simulink model "mrefrobotarm_previous_y_previous_u_previous_ref_cex_3b"  (R2018b)
settings: Solver=FixedStepAuto  StartTime=0.0  StopTime=20  RelTol=1e-3  AbsTol=1e-6
undefined symbols (not defined in the file or in its folder): cc, options
libraries: neural x462, simulink x2
(part 16 of 18)

== system mrefrobotarm_previous_y_previous_u_previous_ref_cex_3b/no_cex/Layer 3/Delays 1 ==
  "p{3}" : Inport  PortDimensions=30
      mask Display: e = 0.06;c1 = [120 230 180]/255;c2 = ([120 230 180]+0)/(256+128);c3 = ([120 230 180]+128)/(256+128);patch([0 1 1 0],[0 0 1 1],c1);patch([0 1 1 1-e 1-e 0+e],[0 0 1 1-e 0+e 0+e],c2);patch([0 0 1 1-e 0+e 0+e],[0 1 1 1-e 1-e 0+e],c3);plot([0 1 1 0 0],[0 0 1 1 0]);
  mux : Mux  Inputs=1
      mask Display: e = 0.06;c1 = [120 150 230]/255;c2 = ([120 150 230]+0)/383;c3 = ([120 150 230]+128)/383;patch([0 1 1 0],[0 0 1 1],c1);patch([0 1 1 1-e 1-e 0+e],[0 0 1 1-e 0+e 0+e],c2);patch([0 0 1 1-e 0+e 0+e],[0 1 1 1-e 1-e 0+e],c3);plot([0 1 1 0 0],[0 0 1 1 0]);disp('Mux')
  "pd{3,2}" : Outport
      mask Display: e = 0.06;c1 = [120 230 180]/255;c2 = ([120 230 180]+0)/(256+128);c3 = ([120 230 180]+128)/(256+128);patch([0 1 1 0],[0 0 1 1],c1);patch([0 1 1 1-e 1-e 0+e],[0 0 1 1-e 0+e 0+e],c2);patch([0 0 1 1-e 0+e 0+e],[0 1 1 1-e 1-e 0+e],c3);plot([0 1 1 0 0],[0 0 1 1 0]);
  wires:
  "p{3}"/1 -> mux/1
  mux/1 -> "pd{3,2}"/1

== system mrefrobotarm_previous_y_previous_u_previous_ref_cex_3b/no_cex/Layer 3/LW{3,2} ==
  "ad{3,2}" : Inport  PortDimensions=30
      mask Display: e = 0.06;c1 = [120 230 180]/255;c2 = ([120 230 180]+0)/(256+128);c3 = ([120 230 180]+128)/(256+128);patch([0 1 1 0],[0 0 1 1],c1);patch([0 1 1 1-e 1-e 0+e],[0 0 1 1-e 0+e 0+e],c2);patch([0 0 1 1-e 0+e 0+e],[0 1 1 1-e 1-e 0+e],c3);plot([0 1 1 0 0],[0 0 1 1 0]);
  "IW{3,2}(1,:)'" : Constant  Value=[-0.055044119527404726521790934157252195291221141815185546875;-0.328920591070812451395255493480362929403781890869140625;0.415372619414880739352469163350178860127925872802734375;-0.228280394241074768846289089196943677961826324462890625;0.16685877262507620155673748740809969604015350341796875;-0.28767716315785907266189269648748449981212615966796875;-0.32128097238228281451455359274405054748058319091796875;0.1207208021741804360171812504631816409528255462646484375;-0.01460580260399220453582103118606028147041797637939453125;0.50165908559916350117902084093657322227954864501953125;0.35772322215377549969872461588238365948200225830078125;-0.00629781978787156970778227105256519280374050140380859375;-0.045079348120089589302406096749109565280377864837646484375;0.00997084703321709196754962789555065683089196681976318359375;0.28527054426915376961204628969426266849040985107421875;0.249132491312471116007287719185114838182926177978515625;-0.1838303477417790876558001400553621351718902587890625;0.4598700488107703154838645787094719707965850830078125;0.0369702760794284046586000158640672452747821807861328125;0.038819346858363877605935243764179176650941371917724609375;0.3202062144887756200972717124386690557003021240234375;-0.022206955571550758554710824910216615535318851470947265625;0.1764209554328330098460497765699983574450016021728515625;-0.369049855517247060721075513356481678783893585205078125;-0.0296667490766724904760476277942871092818677425384521484375;-0.0365536479267042080376626245197257958352565765380859375;0.278066415559107327215571103806723840534687042236328125;0.55989740946528510079360785312019288539886474609375;-0.217843605833106190861059303642832674086093902587890625;0.4063996140330810025176333510898984968662261962890625]
      mask Display: e = 0.06;c1 = [120 150 230]/255;c2 = ([120 150 230]+0)/383;c3 = ([120 150 230]+128)/383;patch([0 1 1 0],[0 0 1 1],c1);patch([0 1 1 1-e 1-e 0+e],[0 0 1 1-e 0+e 0+e],c2);patch([0 0 1 1-e 0+e 0+e],[0 1 1 1-e 1-e 0+e],c3);plot([0 1 1 0 0],[0 0 1 1 0]);disp('weights');
  Mux : Mux  Inputs=1
      mask Display: e = 0.06;c1 = [120 150 230]/255;c2 = ([120 150 230]+0)/383;c3 = ([120 150 230]+128)/383;patch([0 1 1 0],[0 0 1 1],c1);patch([0 1 1 1-e 1-e 0+e],[0 0 1 1-e 0+e 0+e],c2);patch([0 0 1 1-e 0+e 0+e],[0 1 1 1-e 1-e 0+e],c3);plot([0 1 1 0 0],[0 0 1 1 0]);disp('Mux');
  dotprod1 : neural/Weight Functions/dotprod
  "lz{3,2}" : Outport
      mask Display: e = 0.06;c1 = [120 230 180]/255;c2 = ([120 230 180]+0)/(256+128);c3 = ([120 230 180]+128)/(256+128);patch([0 1 1 0],[0 0 1 1],c1);patch([0 1 1 1-e 1-e 0+e],[0 0 1 1-e 0+e 0+e],c2);patch([0 0 1 1-e 0+e 0+e],[0 1 1 1-e 1-e 0+e],c3);plot([0 1 1 0 0],[0 0 1 1 0]);
  wires:
  "IW{3,2}(1,:)'"/1 -> dotprod1/1
  "ad{3,2}"/1 -> dotprod1/2
  dotprod1/1 -> Mux/1
  Mux/1 -> "lz{3,2}"/1

== system mrefrobotarm_previous_y_previous_u_previous_ref_cex_3b/no_cex_15000/Layer 1/Delays 1 ==
  "p{1}" : Inport  PortDimensions=10
      mask Display: e = 0.06;c1 = [120 230 180]/255;c2 = ([120 230 180]+0)/(256+128);c3 = ([120 230 180]+128)/(256+128);patch([0 1 1 0],[0 0 1 1],c1);patch([0 1 1 1-e 1-e 0+e],[0 0 1 1-e 0+e 0+e],c2);patch([0 0 1 1-e 0+e 0+e],[0 1 1 1-e 1-e 0+e],c3);plot([0 1 1 0 0],[0 0 1 1 0]);
  mux : Mux  Inputs=1
      mask Display: e = 0.06;c1 = [120 150 230]/255;c2 = ([120 150 230]+0)/383;c3 = ([120 150 230]+128)/383;patch([0 1 1 0],[0 0 1 1],c1);patch([0 1 1 1-e 1-e 0+e],[0 0 1 1-e 0+e 0+e],c2);patch([0 0 1 1-e 0+e 0+e],[0 1 1 1-e 1-e 0+e],c3);plot([0 1 1 0 0],[0 0 1 1 0]);disp('Mux')
  "pd{1,1}" : Outport
      mask Display: e = 0.06;c1 = [120 230 180]/255;c2 = ([120 230 180]+0)/(256+128);c3 = ([120 230 180]+128)/(256+128);patch([0 1 1 0],[0 0 1 1],c1);patch([0 1 1 1-e 1-e 0+e],[0 0 1 1-e 0+e 0+e],c2);patch([0 0 1 1-e 0+e 0+e],[0 1 1 1-e 1-e 0+e],c3);plot([0 1 1 0 0],[0 0 1 1 0]);
  wires:
  "p{1}"/1 -> mux/1
  mux/1 -> "pd{1,1}"/1

== system mrefrobotarm_previous_y_previous_u_previous_ref_cex_3b/no_cex_15000/Layer 1/IW{1,1} ==
  "pd{1,1}" : Inport  PortDimensions=10
      mask Display: e = 0.06;c1 = [120 230 180]/255;c2 = ([120 230 180]+0)/(256+128);c3 = ([120 230 180]+128)/(256+128);patch([0 1 1 0],[0 0 1 1],c1);patch([0 1 1 1-e 1-e 0+e],[0 0 1 1-e 0+e 0+e],c2);patch([0 0 1 1-e 0+e 0+e],[0 1 1 1-e 1-e 0+e],c3);plot([0 1 1 0 0],[0 0 1 1 0]);
  "IW{1,1}(1,:)'" : Constant  Value=[1.3188511834995317872909481593524105846881866455078125;0.1689480064871527187353450472073745913803577423095703125;0.62298389676086063371229784024762921035289764404296875;-0.39415218427752141128195262353983707726001739501953125;-1.5063673389761664811459240809199400246143341064453125;0.50937741333875352633953070835559628903865814208984375;0.32241543481989853869862372448551468551158905029296875;-0.335387271762626670845719445424037985503673553466796875;-0.58355235109725145381531774546601809561252593994140625;-0.7762464783952396363275738622178323566913604736328125]
      mask Display: e = 0.06;c1 = [120 150 230]/255;c2 = ([120 150 230]+0)/383;c3 = ([120 150 230]+128)/383;patch([0 1 1 0],[0 0 1 1],c1);patch([0 1 1 1-e 1-e 0+e],[0 0 1 1-e 0+e 0+e],c2);patch([0 0 1 1-e 0+e 0+e],[0 1 1 1-e 1-e 0+e],c3);plot([0 1 1 0 0],[0 0 1 1 0]);disp('Weights');
  "IW{1,1}(10,:)'" : Constant  Value=[0.7258859937732449196801098878495395183563232421875;0.2198238550287085202317172161201597191393375396728515625;-0.8129477677772023458402372853015549480915069580078125;0.33409670991292717001641676688450388610363006591796875;0.0762009301501332669825927723650238476693630218505859375;-0.82337222475456883774569405431975610554218292236328125;-0.2019297950314020706485962364240549504756927490234375;-0.88894889200459825673306113458238542079925537109375;2.436157192480757682773173655732534825801849365234375;1.0058276487454878012073322679498232901096343994140625]
      mask Display: e = 0.06;c1 = [120 150 230]/255;c2 = ([120 150 230]+0)/383;c3 = ([120 150 230]+128)/383;patch([0 1 1 0],[0 0 1 1],c1);patch([0 1 1 1-e 1-e 0+e],[0 0 1 1-e 0+e 0+e],c2);patch([0 0 1 1-e 0+e 0+e],[0 1 1 1-e 1-e 0+e],c3);plot([0 1 1 0 0],[0 0 1 1 0]);disp('Weights');
  "IW{1,1}(11,:)'" : Constant  Value=[-0.329810980731012393096790447089006192982196807861328125;0.4709000776860030601511653003399260342121124267578125;-0.98003410643667676627188711790950037539005279541015625;-0.87082647230757237455378572121844626963138580322265625;0.277016665627538072325108942095539532601833343505859375;-0.62337730541465308231607878042268566787242889404296875;0.7378401075831104716229447149089537560939788818359375;-0.436280563315827374371025371146970428526401519775390625;-0.6186629749781584752810204008710570633411407470703125;-0.7776858363996261847006508105550892651081085205078125]
      mask Display: e = 0.06;c1 = [120 150 230]/255;c2 = ([120 150 230]+0)/383;c3 = ([120 150 230]+128)/383;patch([0 1 1 0],[0 0 1 1],c1);patch([0 1 1 1-e 1-e 0+e],[0 0 1 1-e 0+e 0+e],c2);patch([0 0 1 1-e 0+e 0+e],[0 1 1 1-e 1-e 0+e],c3);plot([0 1 1 0 0],[0 0 1 1 0]);disp('Weights');
  "IW{1,1}(12,:)'" : Constant  Value=[0.53957951436292883595768898885580711066722869873046875;-0.55367319387039370948144778594723902642726898193359375;-1.067806415094755490002853548503480851650238037109375;-0.314790535031305107604993054337683133780956268310546875;-0.0301903113325120535381795860985221224837005138397216796875;-0.79597972460447252718296340390224941074848175048828125;0.9233408613690290422937323455698788166046142578125;0.28002836652928431160347599870874546468257904052734375;-0.612473068190372060826121014542877674102783203125;0.15412925045282188651896149167441762983798980712890625]
      mask Display: e = 0.06;c1 = [120 150 230]/255;c2 = ([120 150 230]+0)/383;c3 = ([120 150 230]+128)/383;patch([0 1 1 0],[0 0 1 1],c1);patch([0 1 1 1-e 1-e 0+e],[0 0 1 1-e 0+e 0+e],c2);patch([0 0 1 1-e 0+e 0+e],[0 1 1 1-e 1-e 0+e],c3);plot([0 1 1 0 0],[0 0 1 1 0]);disp('Weights');
  "IW{1,1}(13,:)'" : Constant  Value=[-0.007549105306197079374996850020806959946639835834503173828125;0.59264210166261055423575498934951610863208770751953125;-1.1503522427627166369035194293246604502201080322265625;0.462568606233602130917148542721406556665897369384765625;-0.17257805815617188738286813531885854899883270263671875;0.64446689676790158696206844979315064847469329833984375;-0.1690380289985726758317241547047160565853118896484375;-0.55825379012550324642205623604240827262401580810546875;-1.313955467045924141444857013993896543979644775390625;-0.76754440805176094020367827397421933710575103759765625]
      mask Display: e = 0.06;c1 = [120 150 230]/255;c2 = ([120 150 230]+0)/383;c3 = ([120 150 230]+128)/383;patch([0 1 1 0],[0 0 1 1],c1);patch([0 1 1 1-e 1-e 0+e],[0 0 1 1-e 0+e 0+e],c2);patch([0 0 1 1-e 0+e 0+e],[0 1 1 1-e 1-e 0+e],c3);plot([0 1 1 0 0],[0 0 1 1 0]);disp('Weights');
  "IW{1,1}(14,:)'" : Constant  Value=[0.28879437950909914167851866295677609741687774658203125;0.309031337007359019342089823112473823130130767822265625;0.35490953690414117627227597040473483502864837646484375;0.44617557915201933038673587361699901521205902099609375;-0.817158931264831966956307951477356255054473876953125;-0.631792498376267275261852773837745189666748046875;-0.78411392315008521247676753773703239858150482177734375;0.57409330632700716900984616586356423795223236083984375;0.78284637315219562925250329499249346554279327392578125;-1.07999096319560639045675998204387724399566650390625]
      mask Display: e = 0.06;c1 = [120 150 230]/255;c2 = ([120 150 230]+0)/383;c3 = ([120 150 230]+128)/383;patch([0 1 1 0],[0 0 1 1],c1);patch([0 1 1 1-e 1-e 0+e],[0 0 1 1-e 0+e 0+e],c2);patch([0 0 1 1-e 0+e 0+e],[0 1 1 1-e 1-e 0+e],c3);plot([0 1 1 0 0],[0 0 1 1 0]);disp('Weights');
  "IW{1,1}(15,:)'" : Constant  Value=[-0.2265915888454878845958972988228197209537029266357421875;0.52512734507735758793245395281701348721981048583984375;-0.237067451495421244178629649468348361551761627197265625;-0.50711573329694614731266710805357433855533599853515625;0.53852671039054500479181797345518134534358978271484375;-0.58079797081326611785101476925774477422237396240234375;0.995671396692161092545347855775617063045501708984375;-0.93945924504259947784845508067519403994083404541015625;-1.025726388686293066854204880655743181705474853515625;-0.38905464320706872882738025509752333164215087890625]
      mask Display: e = 0.06;c1 = [120 150 230]/255;c2 = ([120 150 230]+0)/383;c3 = ([120 150 230]+128)/383;patch([0 1 1 0],[0 0 1 1],c1);patch([0 1 1 1-e 1-e 0+e],[0 0 1 1-e 0+e 0+e],c2);patch([0 0 1 1-e 0+e 0+e],[0 1 1 1-e 1-e 0+e],c3);plot([0 1 1 0 0],[0 0 1 1 0]);disp('Weights');
  "IW{1,1}(16,:)'" : Constant  Value=[-0.0999221466547733638829953406457207165658473968505859375;0.58666448347591571010894995197304524481296539306640625;0.38727263657233290672365910722874104976654052734375;-1.063470901218607878035982139408588409423828125;-0.51664598743441902950479516221093945205211639404296875;0.2823348550820128366467542946338653564453125;1.1755784087792588987753106266609393060207366943359375;-0.3872581958704384152980537692201323807239532470703125;-1.157082121110430517063605293515138328075408935546875;-0.139943189411582846748416386617464013397693634033203125]
      mask Display: e = 0.06;c1 = [120 150 230]/255;c2 = ([120 150 230]+0)/383;c3 = ([120 150 230]+128)/383;patch([0 1 1 0],[0 0 1 1],c1);patch([0 1 1 1-e 1-e 0+e],[0 0 1 1-e 0+e 0+e],c2);patch([0 0 1 1-e 0+e 0+e],[0 1 1 1-e 1-e 0+e],c3);plot([0 1 1 0 0],[0 0 1 1 0]);disp('Weights');
  "IW{1,1}(17,:)'" : Constant  Value=[-1.0544613667363627040884921370889060199260711669921875;0.6374843527493412320694687878130935132503509521484375;0.97204043851132926334912554011680185794830322265625;-0.274445558941189549084782584031927399337291717529296875;0.9274982506883187038937421675655059516429901123046875;0.19009005111364007944985132780857384204864501953125;0.027396061293501160205376976364277652464807033538818359375;-0.540807469698680431946513635921292006969451904296875;0.734973254336283243759453398524783551692962646484375;0.0732270695248722625070314506956492550671100616455078125]
      mask Display: e = 0.06;c1 = [120 150 230]/255;c2 = ([120 150 230]+0)/383;c3 = ([120 150 230]+128)/383;patch([0 1 1 0],[0 0 1 1],c1);patch([0 1 1 1-e 1-e 0+e],[0 0 1 1-e 0+e 0+e],c2);patch([0 0 1 1-e 0+e 0+e],[0 1 1 1-e 1-e 0+e],c3);plot([0 1 1 0 0],[0 0 1 1 0]);disp('Weights');
  "IW{1,1}(18,:)'" : Constant  Value=[-0.89871188234364229874273632958647795021533966064453125;0.42025395912304130963121906461310572922229766845703125;0.58890374741419082571525223102071322500705718994140625;-0.151847927074339750230791423746268264949321746826171875;0.3710207290553653169951076051802374422550201416015625;-1.1704828621101786012559387017972767353057861328125;-0.7090359319674470750527461859746836125850677490234375;-0.704089163562461095580147230066359043121337890625;0.93429805546134458982265869053662754595279693603515625;-0.429013324883340541049392413697205483913421630859375]
      mask Display: e = 0.06;c1 = [120 150 230]/255;c2 = ([120 150 230]+0)/383;c3 = ([120 150 230]+128)/383;patch([0 1 1 0],[0 0 1 1],c1);patch([0 1 1 1-e 1-e 0+e],[0 0 1 1-e 0+e 0+e],c2);patch([0 0 1 1-e 0+e 0+e],[0 1 1 1-e 1-e 0+e],c3);plot([0 1 1 0 0],[0 0 1 1 0]);disp('Weights');
  "IW{1,1}(19,:)'" : Constant  Value=[-0.417001732624218579559283170965500175952911376953125;0.98707344091588267165349179776967503130435943603515625;0.4898614856782617099639765001484192907810211181640625;0.45330630838667540505326769562088884413242340087890625;-0.1299710110415610575529399284278042614459991455078125;1.021643488760712426000054620089940726757049560546875;-0.4031698534726906313352401411975733935832977294921875;1.2021287017069113289835513569414615631103515625;-0.01615531649441670491995637348736636340618133544921875;1.3433185622071750486838936922140419483184814453125]
      mask Display: e = 0.06;c1 = [120 150 230]/255;c2 = ([120 150 230]+0)/383;c3 = ([120 150 230]+128)/383;patch([0 1 1 0],[0 0 1 1],c1);patch([0 1 1 1-e 1-e 0+e],[0 0 1 1-e 0+e 0+e],c2);patch([0 0 1 1-e 0+e 0+e],[0 1 1 1-e 1-e 0+e],c3);plot([0 1 1 0 0],[0 0 1 1 0]);disp('Weights');
  "IW{1,1}(2,:)'" : Constant  Value=[-0.50554230655408594063970895149395801126956939697265625;0.384244652236518380306051767547614872455596923828125;0.134351242633984124807966509251855313777923583984375;-0.9758876693323299544857718501589260995388031005859375;0.77057626901546283360033839926472865045070648193359375;-0.6210264607574538242573680690838955342769622802734375;-0.88794546016736575211325543932616710662841796875;0.43376182753206704578730068533332087099552154541015625;1.630690765442163847609435833874158561229705810546875;-0.7186951779849461985349989845417439937591552734375]
      mask Display: e = 0.06;c1 = [120 150 230]/255;c2 = ([120 150 230]+0)/383;c3 = ([120 150 230]+128)/383;patch([0 1 1 0],[0 0 1 1],c1);patch([0 1 1 1-e 1-e 0+e],[0 0 1 1-e 0+e 0+e],c2);patch([0 0 1 1-e 0+e 0+e],[0 1 1 1-e 1-e 0+e],c3);plot([0 1 1 0 0],[0 0 1 1 0]);disp('Weights');
  "IW{1,1}(20,:)'" : Constant  Value=[0.369175002259144735550222549136378802359104156494140625;0.035656774019464508584942308289100765250623226165771484375;-0.43793802030455630802663335998659022152423858642578125;1.2862840722993613695734893553890287876129150390625;0.63014194571868831218353079748339951038360595703125;0.427199716929548778399094999258522875607013702392578125;0.08324862615364732321143748094982584007084369659423828125;0.010629606645243032392311732792222755961120128631591796875;1.4346692081959055986573048357968218624591827392578125;0.949244101443686982833014553762041032314300537109375]
      mask Display: e = 0.06;c1 = [120 150 230]/255;c2 = ([120 150 230]+0)/383;c3 = ([120 150 230]+128)/383;patch([0 1 1 0],[0 0 1 1],c1);patch([0 1 1 1-e 1-e 0+e],[0 0 1 1-e 0+e 0+e],c2);patch([0 0 1 1-e 0+e 0+e],[0 1 1 1-e 1-e 0+e],c3);plot([0 1 1 0 0],[0 0 1 1 0]);disp('Weights');
  "IW{1,1}(21,:)'" : Constant  Value=[-0.1520499106373587039353623140414129011332988739013671875;0.8567201387698519798874485786654986441135406494140625;-0.553451704659411181097539156326092779636383056640625;1.0619758955597633498513232552795670926570892333984375;0.07790635762702909083987634630830143578350543975830078125;0.018719652245145775026902157378572155721485614776611328125;0.3007721816297959094299585558474063873291015625;1.0136655538582497459998421618365682661533355712890625;-0.52169208072516026764020580230862833559513092041015625;1.0309770572411600664253228387678973376750946044921875]
      mask Display: e = 0.06;c1 = [120 150 230]/255;c2 = ([120 150 230]+0)/383;c3 = ([120 150 230]+128)/383;patch([0 1 1 0],[0 0 1 1],c1);patch([0 1 1 1-e 1-e 0+e],[0 0 1 1-e 0+e 0+e],c2);patch([0 0 1 1-e 0+e 0+e],[0 1 1 1-e 1-e 0+e],c3);plot([0 1 1 0 0],[0 0 1 1 0]);disp('Weights');
  "IW{1,1}(22,:)'" : Constant  Value=[-0.85240004634796140425834209963795728981494903564453125;-0.09223424224898636725189504659283556975424289703369140625;-0.173437645673212570418542100014747120440006256103515625;-0.08848165837472306283206791022166726179420948028564453125;-0.89053817966496395808206898436765186488628387451171875;-0.2281182231841629715063390904106199741363525390625;0.48704057905408759676646468506078235805034637451171875;0.462402350219965285749168515394558198750019073486328125;-0.87912063081110936035855729642207734286785125732421875;-0.170058966547850631823024514233111403882503509521484375]
      mask Display: e = 0.06;c1 = [120 150 230]/255;c2 = ([120 150 230]+0)/383;c3 = ([120 150 230]+128)/383;patch([0 1 1 0],[0 0 1 1],c1);patch([0 1 1 1-e 1-e 0+e],[0 0 1 1-e 0+e 0+e],c2);patch([0 0 1 1-e 0+e 0+e],[0 1 1 1-e 1-e 0+e],c3);plot([0 1 1 0 0],[0 0 1 1 0]);disp('Weights');
  "IW{1,1}(23,:)'" : Constant  Value=[-0.2046809124756551467871901195394457317888736724853515625;0.257591221065810727086642373251379467546939849853515625;-0.1100426723887848456939764218986965715885162353515625;-0.8825833917260457184283950482495129108428955078125;0.50573874113278305397756184902391396462917327880859375;-0.407327619285202668919509960687719285488128662109375;0.0279488291136463819219759585621432051993906497955322265625;0.58860086469138461762184988401713781058788299560546875;-2.178257009849004166568420259864069521427154541015625;-0.92021942608696460919048831783584319055080413818359375]
      mask Display: e = 0.06;c1 = [120 150 230]/255;c2 = ([120 150 230]+0)/383;c3 = ([120 150 230]+128)/383;patch([0 1 1 0],[0 0 1 1],c1);patch([0 1 1 1-e 1-e 0+e],[0 0 1 1-e 0+e 0+e],c2);patch([0 0 1 1-e 0+e 0+e],[0 1 1 1-e 1-e 0+e],c3);plot([0 1 1 0 0],[0 0 1 1 0]);disp('Weights');
  "IW{1,1}(24,:)'" : Constant  Value=[0.181013130350561712855750329254078678786754608154296875;-0.79368658000463410129299290929338894784450531005859375;0.6497863163794959096009051791043020784854888916015625;-0.269905248171758593844771212388877756893634796142578125;-0.444655746522254979868904456452582962810993194580078125;1.368472219583368509887577602057717740535736083984375;-0.044488912976583978864386637042116490192711353302001953125;0.216697820325806755903386147110722959041595458984375;0.69899709344569072033692691547912545502185821533203125;-0.1670680902355327346331392845968366600573062896728515625]
      mask Display: e = 0.06;c1 = [120 150 230]/255;c2 = ([120 150 230]+0)/383;c3 = ([120 150 230]+128)/383;patch([0 1 1 0],[0 0 1 1],c1);patch([0 1 1 1-e 1-e 0+e],[0 0 1 1-e 0+e 0+e],c2);patch([0 0 1 1-e 0+e 0+e],[0 1 1 1-e 1-e 0+e],c3);plot([0 1 1 0 0],[0 0 1 1 0]);disp('Weights');
  "IW{1,1}(25,:)'" : Constant  Value=[-0.54672076928667345807610900010331533849239349365234375;-0.3997584174064334749942872804240323603153228759765625;-0.71460399371026539494522467066417448222637176513671875;0.6076905754182087004977574906661175191402435302734375;-0.5468266301868156542553833787678740918636322021484375;0.1365556170579986516866455303897964768111705780029296875;-1.04704081125050141309884565998800098896026611328125;0.6184374571274207088578123148181475698947906494140625;1.6936248461637901652210302927414886653423309326171875;0.93624589617214493131314156926237046718597412109375]
      mask Display: e = 0.06;c1 = [120 150 230]/255;c2 = ([120 150 230]+0)/383;c3 = ([120 150 230]+128)/383;patch([0 1 1 0],[0 0 1 1],c1);patch([0 1 1 1-e 1-e 0+e],[0 0 1 1-e 0+e 0+e],c2);patch([0 0 1 1-e 0+e 0+e],[0 1 1 1-e 1-e 0+e],c3);plot([0 1 1 0 0],[0 0 1 1 0]);disp('Weights');
  "IW{1,1}(26,:)'" : Constant  Value=[-0.86012157461298655025672132978797890245914459228515625;0.12386758869929799520281932245779898948967456817626953125;0.6587136768166050870831895736046135425567626953125;0.03555959427852832532845894775164197199046611785888671875;0.486354306310446904415556446110713295638561248779296875;-0.0802392303934685580113495007026358507573604583740234375;0.631557933480137112525198972434736788272857666015625;0.7617108027674621695268797338940203189849853515625;-2.549822845814477378922902062186039984226226806640625;-1.8830595480469136671075602862401865422725677490234375]
      mask Display: e = 0.06;c1 = [120 150 230]/255;c2 = ([120 150 230]+0)/383;c3 = ([120 150 230]+128)/383;patch([0 1 1 0],[0 0 1 1],c1);patch([0 1 1 1-e 1-e 0+e],[0 0 1 1-e 0+e 0+e],c2);patch([0 0 1 1-e 0+e 0+e],[0 1 1 1-e 1-e 0+e],c3);plot([0 1 1 0 0],[0 0 1 1 0]);disp('Weights');
  "IW{1,1}(27,:)'" : Constant  Value=[-1.9273960362381610256221620147698558866977691650390625;-0.50123696817146823345723305465071462094783782958984375;-0.3815024762727874385603854534565471112728118896484375;1.040175531592041568984541299869306385517120361328125;0.99583272840992587138231328935944475233554840087890625;0.07855815699580770417043140696478076279163360595703125;0.6500224149843958354466622040490619838237762451171875;-0.94371686548830524543518549762666225433349609375;0.87080721810348060696327365803881548345088958740234375;1.8318024165726143337451503612101078033447265625]
      mask Display: e = 0.06;c1 = [120 150 230]/255;c2 = ([120 150 230]+0)/383;c3 = ([120 150 230]+128)/383;patch([0 1 1 0],[0 0 1 1],c1);patch([0 1 1 1-e 1-e 0+e],[0 0 1 1-e 0+e 0+e],c2);patch([0 0 1 1-e 0+e 0+e],[0 1 1 1-e 1-e 0+e],c3);plot([0 1 1 0 0],[0 0 1 1 0]);disp('Weights');
  "IW{1,1}(28,:)'" : Constant  Value=[-1.1064247952049643952676660774159245193004608154296875;0.2260329278664475471938288819728768430650234222412109375;0.263333634055948617724851601451518945395946502685546875;-0.194848016842403215509449410092202015221118927001953125;-1.23077374276916540196680216467939317226409912109375;-0.1371783337140443925772359534676070325076580047607421875;0.08789441640293439717002144107027561403810977935791015625;-0.0988911483319735162833552521988167427480220794677734375;-0.1019287494032759811002364358500926755368709564208984375;0.3374325274750535896828296245075762271881103515625]
      mask Display: e = 0.06;c1 = [120 150 230]/255;c2 = ([120 150 230]+0)/383;c3 = ([120 150 230]+128)/383;patch([0 1 1 0],[0 0 1 1],c1);patch([0 1 1 1-e 1-e 0+e],[0 0 1 1-e 0+e 0+e],c2);patch([0 0 1 1-e 0+e 0+e],[0 1 1 1-e 1-e 0+e],c3);plot([0 1 1 0 0],[0 0 1 1 0]);disp('Weights');
  "IW{1,1}(29,:)'" : Constant  Value=[0.67864438920905201246824844929506070911884307861328125;-0.84873715178308095641313002488459460437297821044921875;0.759745880061066802824143451289273798465728759765625;1.34270229039540112125905579887330532073974609375;-0.03064054730453870389883519465001882053911685943603515625;0.036135199499689178714856296892321552149951457977294921875;1.0446922125858073560067396101658232510089874267578125;0.05192716264434703299368578655048622749745845794677734375;0.0259983433134954346199751995527549297548830509185791015625;0.383228269174186564338668858908931724727153778076171875]
      mask Display: e = 0.06;c1 = [120 150 230]/255;c2 = ([120 150 230]+0)/383;c3 = ([120 150 230]+128)/383;patch([0 1 1 0],[0 0 1 1],c1);patch([0 1 1 1-e 1-e 0+e],[0 0 1 1-e 0+e 0+e],c2);patch([0 0 1 1-e 0+e 0+e],[0 1 1 1-e 1-e 0+e],c3);plot([0 1 1 0 0],[0 0 1 1 0]);disp('Weights');
  "IW{1,1}(3,:)'" : Constant  Value=[0.2486311695592009207711470253343577496707439422607421875;0.636745498382498720246758239227347075939178466796875;-0.271672841742817638976958960483898408710956573486328125;0.334143158234913972837176743269083090126514434814453125;0.7932820169693581835446138939005322754383087158203125;-0.41075609729863005181726975933997891843318939208984375;1.0223078977324477900623378445743583142757415771484375;0.657939429804926145806120985071174800395965576171875;0.560000067505167731241044748458079993724822998046875;1.086407957673689583799614410963840782642364501953125]
      mask Display: e = 0.06;c1 = [120 150 230]/255;c2 = ([120 150 230]+0)/383;c3 = ([120 150 230]+128)/383;patch([0 1 1 0],[0 0 1 1],c1);patch([0 1 1 1-e 1-e 0+e],[0 0 1 1-e 0+e 0+e],c2);patch([0 0 1 1-e 0+e 0+e],[0 1 1 1-e 1-e 0+e],c3);plot([0 1 1 0 0],[0 0 1 1 0]);disp('Weights');
  "IW{1,1}(30,:)'" : Constant  Value=[1.45995008180757945837058286997489631175994873046875;0.71700011926277096296900026572984643280506134033203125;-0.53351478941311381021250781486742198467254638671875;-0.1909653784829092870722888619638979434967041015625;-0.147236378283638169595093359021120704710483551025390625;-1.21675540926733294355699399602599442005157470703125;0.87989668820765698509234198354533873498439788818359375;0.541883892139802814114091233932413160800933837890625;-1.3016496093540899092744211884564720094203948974609375;-0.7668645609230129167599443462677299976348876953125]
      mask Display: e = 0.06;c1 = [120 150 230]/255;c2 = ([120 150 230]+0)/383;c3 = ([120 150 230]+128)/383;patch([0 1 1 0],[0 0 1 1],c1);patch([0 1 1 1-e 1-e 0+e],[0 0 1 1-e 0+e 0+e],c2);patch([0 0 1 1-e 0+e 0+e],[0 1 1 1-e 1-e 0+e],c3);plot([0 1 1 0 0],[0 0 1 1 0]);disp('Weights');
  "IW{1,1}(4,:)'" : Constant  Value=[0.0764367863716351181313513052373309619724750518798828125;-0.0194119811502705304218086013179345172829926013946533203125;-0.50785137238099131717916634443099610507488250732421875;0.69326201445987745142218727778526954352855682373046875;-0.25720636416341513541539143261616118252277374267578125;1.080325572156194180450938802096061408519744873046875;-0.365292214522681402133486017191899009048938751220703125;0.196725891690471554884567240151227451860904693603515625;1.6372199993449243482501742619206197559833526611328125;0.378775473354196645647817831559223122894763946533203125]
      mask Display: e = 0.06;c1 = [120 150 230]/255;c2 = ([120 150 230]+0)/383;c3 = ([120 150 230]+128)/383;patch([0 1 1 0],[0 0 1 1],c1);patch([0 1 1 1-e 1-e 0+e],[0 0 1 1-e 0+e 0+e],c2);patch([0 0 1 1-e 0+e 0+e],[0 1 1 1-e 1-e 0+e],c3);plot([0 1 1 0 0],[0 0 1 1 0]);disp('Weights');
  "IW{1,1}(5,:)'" : Constant  Value=[-0.28777637039310743904962919259560294449329376220703125;-0.9326589328964747238615018432028591632843017578125;-0.31940294675014302416826694752671755850315093994140625;-2.5891106010402875625686647254042327404022216796875;-0.82258004156175801302453010066528804600238800048828125;-1.0623229341430562300274687004275619983673095703125;0.96137681933998930805529425924760289490222930908203125;-1.567743300823500884888517248327843844890594482421875;-1.823512942172554662789707435877062380313873291015625;-1.2165834101861567884128589867032133042812347412109375]
      mask Display: e = 0.06;c1 = [120 150 230]/255;c2 = ([120 150 230]+0)/383;c3 = ([120 150 230]+128)/383;patch([0 1 1 0],[0 0 1 1],c1);patch([0 1 1 1-e 1-e 0+e],[0 0 1 1-e 0+e 0+e],c2);patch([0 0 1 1-e 0+e 0+e],[0 1 1 1-e 1-e 0+e],c3);plot([0 1 1 0 0],[0 0 1 1 0]);disp('Weights');
  "IW{1,1}(6,:)'" : Constant  Value=[0.7134550049392214265964184960466809570789337158203125;-0.2166771479933629340752787584278848953545093536376953125;0.8192958266282881485409461674862541258335113525390625;0.369585417764502432991235991721623577177524566650390625;-0.191808936345291447533867312813526950776576995849609375;1.10599335493272388220020729932002723217010498046875;0.1624712178069334378438526300669764168560504913330078125;0.579045327383761243567050769343040883541107177734375;-0.09700519503648319386002185638062655925750732421875;1.204163156786230981509788762195967137813568115234375]
      mask Display: e = 0.06;c1 = [120 150 230]/255;c2 = ([120 150 230]+0)/383;c3 = ([120 150 230]+128)/383;patch([0 1 1 0],[0 0 1 1],c1);patch([0 1 1 1-e 1-e 0+e],[0 0 1 1-e 0+e 0+e],c2);patch([0 0 1 1-e 0+e 0+e],[0 1 1 1-e 1-e 0+e],c3);plot([0 1 1 0 0],[0 0 1 1 0]);disp('Weights');
  "IW{1,1}(7,:)'" : Constant  Value=[0.293554095299895845272430960903875529766082763671875;1.3634226909240556580016345833428204059600830078125;-0.09436536861101922635253202997773769311606884002685546875;1.0980466798536692163423822421464137732982635498046875;1.106813871987203157232215744443237781524658203125;-0.55289240323160526724421970357070676982402801513671875;0.93929543125915415657800622284412384033203125;1.650296510299666952192865210236050188541412353515625;-0.258959314122750805520212225019349716603755950927734375;0.351264446917976869144695228897035121917724609375]
      mask Display: e = 0.06;c1 = [120 150 230]/255;c2 = ([120 150 230]+0)/383;c3 = ([120 150 230]+128)/383;patch([0 1 1 0],[0 0 1 1],c1);patch([0 1 1 1-e 1-e 0+e],[0 0 1 1-e 0+e 0+e],c2);patch([0 0 1 1-e 0+e 0+e],[0 1 1 1-e 1-e 0+e],c3);plot([0 1 1 0 0],[0 0 1 1 0]);disp('Weights');
  "IW{1,1}(8,:)'" : Constant  Value=[-0.28851636757948806444318279318395070731639862060546875;1.0964327629942196562495837497408501803874969482421875;-0.6986520017086588207888553370139561593532562255859375;1.05565908284800258343238965608179569244384765625;0.06803319294494848679111242972794570960104465484619140625;-0.1297740726236859265529943741057650186121463775634765625;-0.462546768056460388951478535091155208647251129150390625;0.4154589300888849034976146867848001420497894287109375;0.408227450318047413446720383944921195507049560546875;0.821426641491572961939482411253266036510467529296875]
      mask Display: e = 0.06;c1 = [120 150 230]/255;c2 = ([120 150 230]+0)/383;c3 = ([120 150 230]+128)/383;patch([0 1 1 0],[0 0 1 1],c1);patch([0 1 1 1-e 1-e 0+e],[0 0 1 1-e 0+e 0+e],c2);patch([0 0 1 1-e 0+e 0+e],[0 1 1 1-e 1-e 0+e],c3);plot([0 1 1 0 0],[0 0 1 1 0]);disp('Weights');
  "IW{1,1}(9,:)'" : Constant  Value=[0.027273870132686284240008944834698922932147979736328125;-0.7238349351229473871427444464643485844135284423828125;0.26402932967293535337915955096832476556301116943359375;0.8869147706206883530200002496712841093540191650390625;0.7198378601729908954354186789714731276035308837890625;0.367209660601583942618475475683226250112056732177734375;-0.022568180704131864111605665357274119742214679718017578125;1.0930312680096341271251958460197784006595611572265625;0.25654486040122159717924432698055170476436614990234375;1.4018971598469054384850096539594233036041259765625]
      mask Display: e = 0.06;c1 = [120 150 230]/255;c2 = ([120 150 230]+0)/383;c3 = ([120 150 230]+128)/383;patch([0 1 1 0],[0 0 1 1],c1);patch([0 1 1 1-e 1-e 0+e],[0 0 1 1-e 0+e 0+e],c2);patch([0 0 1 1-e 0+e 0+e],[0 1 1 1-e 1-e 0+e],c3);plot([0 1 1 0 0],[0 0 1 1 0]);disp('Weights');
  Mux : Mux  Inputs=30
      mask Display: e = 0.06;c1 = [120 150 230]/255;c2 = ([120 150 230]+0)/383;c3 = ([120 150 230]+128)/383;patch([0 1 1 0],[0 0 1 1],c1);patch([0 1 1 1-e 1-e 0+e],[0 0 1 1-e 0+e 0+e],c2);patch([0 0 1 1-e 0+e 0+e],[0 1 1 1-e 1-e 0+e],c3);plot([0 1 1 0 0],[0 0 1 1 0]);disp('Mux');
  dotprod{1..30} (30 alike) : neural/Weight Functions/dotprod
  "iz{1,1}" : Outport
      mask Display: e = 0.06;c1 = [120 230 180]/255;c2 = ([120 230 180]+0)/(256+128);c3 = ([120 230 180]+128)/(256+128);patch([0 1 1 0],[0 0 1 1],c1);patch([0 1 1 1-e 1-e 0+e],[0 0 1 1-e 0+e 0+e],c2);patch([0 0 1 1-e 0+e 0+e],[0 1 1 1-e 1-e 0+e],c3);plot([0 1 1 0 0],[0 0 1 1 0]);
  wires:
  "IW{1,1}(1,:)'"/1 -> dotprod1/1
  "pd{1,1}"/1 -> dotprod1/2, dotprod2/2, dotprod3/2, dotprod4/2, dotprod5/2, dotprod6/2, dotprod7/2, dotprod8/2, dotprod9/2, dotprod10/2, dotprod11/2, dotprod12/2, dotprod13/2, dotprod14/2, dotprod15/2, dotprod16/2, dotprod17/2, dotprod18/2, dotprod19/2, dotprod20/2, dotprod21/2, dotprod22/2, dotprod23/2, dotprod24/2, dotprod25/2, dotprod26/2, dotprod27/2, dotprod28/2, dotprod29/2, dotprod30/2
  dotprod1/1 -> Mux/1
  "IW{1,1}(2,:)'"/1 -> dotprod2/1
  dotprod2/1 -> Mux/2
  "IW{1,1}(3,:)'"/1 -> dotprod3/1
  dotprod3/1 -> Mux/3
  "IW{1,1}(4,:)'"/1 -> dotprod4/1
  dotprod4/1 -> Mux/4
  "IW{1,1}(5,:)'"/1 -> dotprod5/1
  dotprod5/1 -> Mux/5
  "IW{1,1}(6,:)'"/1 -> dotprod6/1
  dotprod6/1 -> Mux/6
  "IW{1,1}(7,:)'"/1 -> dotprod7/1
  dotprod7/1 -> Mux/7
  "IW{1,1}(8,:)'"/1 -> dotprod8/1
  dotprod8/1 -> Mux/8
  "IW{1,1}(9,:)'"/1 -> dotprod9/1
  dotprod9/1 -> Mux/9
  "IW{1,1}(10,:)'"/1 -> dotprod10/1
  dotprod10/1 -> Mux/10
  "IW{1,1}(11,:)'"/1 -> dotprod11/1
  dotprod11/1 -> Mux/11
  "IW{1,1}(12,:)'"/1 -> dotprod12/1
  dotprod12/1 -> Mux/12
  "IW{1,1}(13,:)'"/1 -> dotprod13/1
  dotprod13/1 -> Mux/13
  "IW{1,1}(14,:)'"/1 -> dotprod14/1
  dotprod14/1 -> Mux/14
  "IW{1,1}(15,:)'"/1 -> dotprod15/1
  dotprod15/1 -> Mux/15
  "IW{1,1}(16,:)'"/1 -> dotprod16/1
  dotprod16/1 -> Mux/16
  "IW{1,1}(17,:)'"/1 -> dotprod17/1
  dotprod17/1 -> Mux/17
  "IW{1,1}(18,:)'"/1 -> dotprod18/1
  dotprod18/1 -> Mux/18
  "IW{1,1}(19,:)'"/1 -> dotprod19/1
  dotprod19/1 -> Mux/19
  "IW{1,1}(20,:)'"/1 -> dotprod20/1
  dotprod20/1 -> Mux/20
  "IW{1,1}(21,:)'"/1 -> dotprod21/1
  dotprod21/1 -> Mux/21
  "IW{1,1}(22,:)'"/1 -> dotprod22/1
  dotprod22/1 -> Mux/22
  "IW{1,1}(23,:)'"/1 -> dotprod23/1
  dotprod23/1 -> Mux/23
  "IW{1,1}(24,:)'"/1 -> dotprod24/1
  dotprod24/1 -> Mux/24
  "IW{1,1}(25,:)'"/1 -> dotprod25/1
  dotprod25/1 -> Mux/25
  "IW{1,1}(26,:)'"/1 -> dotprod26/1
  dotprod26/1 -> Mux/26
  "IW{1,1}(27,:)'"/1 -> dotprod27/1
  dotprod27/1 -> Mux/27
  "IW{1,1}(28,:)'"/1 -> dotprod28/1
  dotprod28/1 -> Mux/28
  "IW{1,1}(29,:)'"/1 -> dotprod29/1
  dotprod29/1 -> Mux/29
  "IW{1,1}(30,:)'"/1 -> dotprod30/1
  dotprod30/1 -> Mux/30
  Mux/1 -> "iz{1,1}"/1

== system mrefrobotarm_previous_y_previous_u_previous_ref_cex_3b/no_cex_15000/Layer 2/Delays 1 ==
  "p{2}" : Inport  PortDimensions=30
      mask Display: e = 0.06;c1 = [120 230 180]/255;c2 = ([120 230 180]+0)/(256+128);c3 = ([120 230 180]+128)/(256+128);patch([0 1 1 0],[0 0 1 1],c1);patch([0 1 1 1-e 1-e 0+e],[0 0 1 1-e 0+e 0+e],c2);patch([0 0 1 1-e 0+e 0+e],[0 1 1 1-e 1-e 0+e],c3);plot([0 1 1 0 0],[0 0 1 1 0]);
  mux : Mux  Inputs=1
      mask Display: e = 0.06;c1 = [120 150 230]/255;c2 = ([120 150 230]+0)/383;c3 = ([120 150 230]+128)/383;patch([0 1 1 0],[0 0 1 1],c1);patch([0 1 1 1-e 1-e 0+e],[0 0 1 1-e 0+e 0+e],c2);patch([0 0 1 1-e 0+e 0+e],[0 1 1 1-e 1-e 0+e],c3);plot([0 1 1 0 0],[0 0 1 1 0]);disp('Mux')
  "pd{2,1}" : Outport
      mask Display: e = 0.06;c1 = [120 230 180]/255;c2 = ([120 230 180]+0)/(256+128);c3 = ([120 230 180]+128)/(256+128);patch([0 1 1 0],[0 0 1 1],c1);patch([0 1 1 1-e 1-e 0+e],[0 0 1 1-e 0+e 0+e],c2);patch([0 0 1 1-e 0+e 0+e],[0 1 1 1-e 1-e 0+e],c3);plot([0 1 1 0 0],[0 0 1 1 0]);
  wires:
  "p{2}"/1 -> mux/1
  mux/1 -> "pd{2,1}"/1
